simulink model "NewLinearModel"  (R2020b)
settings: Solver=VariableStepAuto  StartTime=0.0  StopTime=1000  RelTol=1e-3
values from neighbouring files (symbols this model uses):
  A_1 = linsys1.A    [AssignMatrices.m]
  B_1 = linsys1.B    [AssignMatrices.m]
  C_1 = linsys1.C    [AssignMatrices.m]
  D_1 = linsys1.D    [AssignMatrices.m]
  u0_Thrust = fileName.Inputs(4).u    [AssignMatrices.m]
  u1max = deg2rad(25)    [AssignMatrices.m]
  u1min = deg2rad(-25)    [AssignMatrices.m]
  u2max = deg2rad(10)    [AssignMatrices.m]
  u2min = deg2rad(-25)    [AssignMatrices.m]
  u3max = deg2rad(30)    [AssignMatrices.m]
  u3min = deg2rad(-30)    [AssignMatrices.m]
undefined symbols (not defined in the file or in its folder): sigbuilder_block
libraries: pid_lib x14, sharedtransform x1, simulink_extras x1
(part 2 of 2)

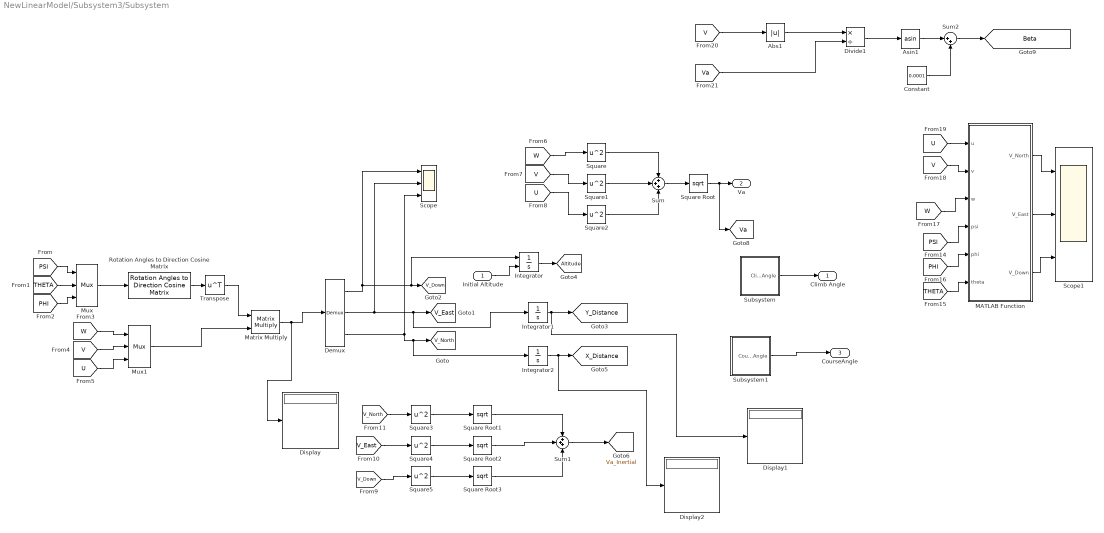
== system NewLinearModel/Subsystem3/Subsystem ==
  Initial Altitude : Inport
  Abs1 : Abs
  Asin1 : Trigonometry  Operator=asin
  Constant : Constant  Value=0.0001
  Demux : Demux  Outputs=3
  Display : Display
  Display1 : Display
  Display2 : Display
  Divide1 : Product  Inputs=*/
  Integrator : Integrator  InitialConditionSource=external  LowerSaturationLimit=0
  Integrator1 : Integrator  UpperSaturationLimit=+10  LowerSaturationLimit=-10
  Integrator2 : Integrator  LimitOutput=on
  MATLAB Function : MATLAB Function  TreatAsAtomicUnit=on
  Matrix Multiply : Product  Multiplication=Matrix(*)
  Mux : Mux  Inputs=3
  Mux1 : Mux  Inputs=3
  Rotation Angles to Direction Cosine Matrix : sharedtransform/Rotation Angles to Direction Cosine Matrix  rotationOrder=ZYX  aMode=aMode
      settings: SourceProductBaseCode=AE,PW,MT,UV,VE,VP
  Scope : Scope  NumInputPorts=3
  Scope1 : Scope  NumInputPorts=3
  Square{,1..5} (6 alike) : Math  Operator=square  SaturateOnIntegerOverflow=on
  Square Root{,1..3} (4 alike) : Sqrt  SaturateOnIntegerOverflow=on
  Subsystem : Subsystem
  Subsystem1 : Subsystem
  Sum : Sum  Inputs=+++
  Sum1 : Sum  Inputs=+++
  Sum2 : Sum  Inputs=|++
  Transpose : Math  Operator=transpose  SignedPower=on  SaturateOnIntegerOverflow=on
  Climb Angle : Outport
  Va : Outport  Port=2
  CourseAngle : Outport  Port=3
  tag scope: Altitude=global, Beta=global, V_Down=global, V_East=global, V_North=global, Va=global, Va_Inertial=global, X_Distance=global, Y_Distance=global
  wires:
  Square1/1 -> Sum/2
  Square Root/1 -> [Va], Va/1
  Sum/1 -> Square Root/1
  Square2/1 -> Sum/3
  Square/1 -> Sum/1
  Subsystem/1(Climb Angle) -> Climb Angle/1
  Rotation Angles to Direction Cosine Matrix/1 -> Transpose/1
  Mux/1 -> Rotation Angles to Direction Cosine Matrix/1
  Transpose/1 -> Matrix Multiply/1
  Mux1/1 -> Matrix Multiply/2
  Matrix Multiply/1 -> Display/1, Demux/1
  Demux/1 -> Integrator/1, [V_Down], Scope/1
  Demux/2 -> Integrator1/1, [V_East], Scope/2
  Demux/3 -> Integrator2/1, [V_North], Scope/3
  [PSI] -> Mux/1
  [PHI] -> Mux/3
  [THETA] -> Mux/2
  [W] -> Mux1/1
  [V] -> Mux1/2
  [U] -> Mux1/3
  [W] -> Square/1
  [V] -> Square1/1
  [U] -> Square2/1
  Subsystem1/1(CourseAngle) -> CourseAngle/1
  Initial Altitude/1 -> Integrator/2
  Integrator1/1 -> Display1/1, [Y_Distance]
  Integrator2/1 -> Display2/1, [X_Distance]
  [V_Down] -> Square5/1
  [V_East] -> Square4/1
  [V_North] -> Square3/1
  Square5/1 -> Square Root3/1
  Square4/1 -> Square Root2/1
  Square3/1 -> Square Root1/1
  Square Root1/1 -> Sum1/1
  Square Root2/1 -> Sum1/2
  Square Root3/1 -> Sum1/3
  Sum1/1 -> [Va_Inertial]
  [PHI] -> MATLAB Function/5(phi)
  [PSI] -> MATLAB Function/4(psi)
  [THETA] -> MATLAB Function/6(theta)
  [U] -> MATLAB Function/1(u)
  [V] -> MATLAB Function/2(v)
  [W] -> MATLAB Function/3(w)
  MATLAB Function/1(V_North) -> Scope1/1
  MATLAB Function/2(V_East) -> Scope1/2
  MATLAB Function/3(V_Down) -> Scope1/3
  Integrator/1 -> [Altitude]
  Abs1/1 -> Divide1/1
  Divide1/1 -> Asin1/1
  [V] -> Abs1/1
  [Va] -> Divide1/2
  Sum2/1 -> [Beta]
  Asin1/1 -> Sum2/1
  Constant/1 -> Sum2/2

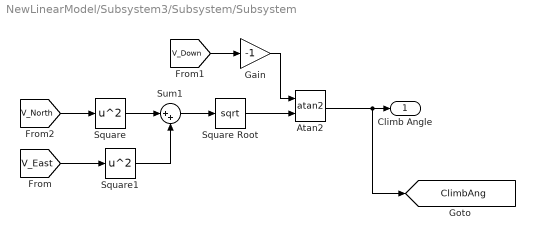
== system NewLinearModel/Subsystem3/Subsystem/Subsystem ==
  Atan2 : Trigonometry  Operator=atan2
  Gain : Gain  Gain=-1
  Square : Math  Operator=square  SaturateOnIntegerOverflow=on
  Square Root : Sqrt  SaturateOnIntegerOverflow=on
  Square1 : Math  Operator=square  SaturateOnIntegerOverflow=on
  Sum1 : Sum  Inputs=|++
  Climb Angle : Outport
  tag scope: ClimbAng=global
  wires:
  Atan2/1 -> [ClimbAng], Climb Angle/1
  [V_North] -> Square/1
  [V_East] -> Square1/1
  Square/1 -> Sum1/1
  Square1/1 -> Sum1/2
  Sum1/1 -> Square Root/1
  Square Root/1 -> Atan2/2
  [V_Down] -> Gain/1
  Gain/1 -> Atan2/1

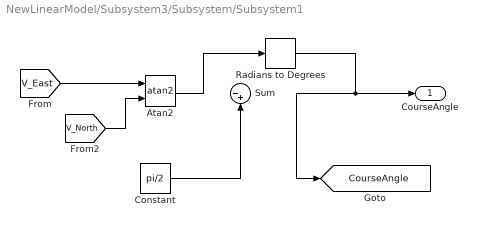
== system NewLinearModel/Subsystem3/Subsystem/Subsystem1 ==
  Atan2 : Trigonometry  Operator=atan2
  Constant : Constant  Value=pi/2
  Radians to Degrees : simulink_extras/Transformations/Radians to Degrees
  Sum : Sum  Inputs=|-+
  CourseAngle : Outport
  tag scope: CourseAngle=global
  wires:
  Constant/1 -> Sum/2
  [V_East] -> Atan2/1
  [V_North] -> Atan2/2
  Atan2/1 -> Radians to Degrees/1
  Radians to Degrees/1 -> [CourseAngle], CourseAngle/1

== matlab function NewLinearModel/Subsystem3/Subsystem/MATLAB Function ==
  data: u input; V_North output; v input; w input; psi input; phi input; theta input; V_East output; V_Down output
function [V_North, V_East, V_Down] = fcn(u,v,w,psi,phi,theta)

% V_North = u*(cos(theta)*cos(psi)) + v*(sin(phi)*sin(theta)*cos(psi)- cos(phi)*sin(psi)) + w*(cos(phi)*sin(theta)*cos(psi)+sin(phi)*sin(psi));
% V_East = u*(cos(theta)*sin(psi)) + v*(sin(phi)*sin(theta)*sin(psi) + cos(phi)*cos(psi)) + w*(cos(phi)*sin(theta)*cos(psi)-sin(phi)*cos(psi));
% V_Down = u*(-sin(theta)) + v*(sin(phi)*cos(theta)) + w*(cos(phi)*cos(theta));

x7 = phi;
x8 = theta;
x9 = psi;

V_b = [u;v;w];

C12 = [cos(x9) -sin(x9) 0;
        sin(x9) cos(x9) 0;
        0 0 1];
C23 = [cos(x8) 0 sin(x8);
        0 1 0;
        -sin(x8) 0 cos(x8)];
C3i = [1 0 0;
    0 cos(x7) -sin(x7);
    0 sin(x7) cos(x7)];


Cvb = C12*C23*C3i; 

V_Earth = Cvb * V_b;

V_North = V_Earth(1);
V_East = V_Earth(2);
V_Down = V_Earth(3);
